simulink model "kalman_predictor"  (R2014a)
settings: Solver=FixedStepDiscrete  StartTime=0.0  StopTime=t_sim  FixedStep=t_step  RelTol=1e-3
undefined symbols (not defined in the file): omega_B
libraries: lib_gyro_fusion x3
settings Model: Creator=kirill  LastModifiedBy=kirill

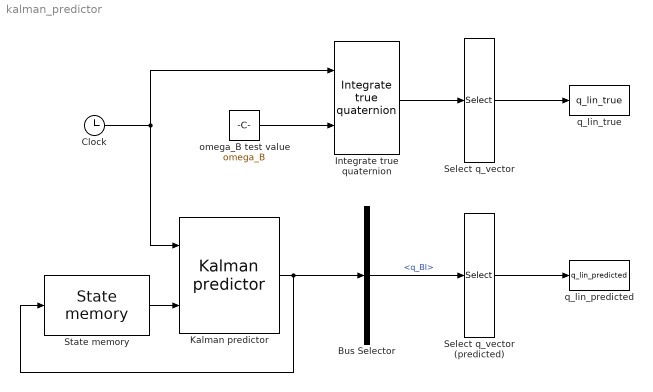
== system kalman_predictor ==
  Bus Selector : BusSelector  OutputSignals=q_BI
  Clock : Clock
  Integrate true quaternion : lib_gyro_fusion/Integrate true quaternion  q_BI_init=q_init
  Kalman predictor : lib_gyro_fusion/Kalman predictor  q_noise=0  omega_B_noise=[0, 0, 0]  omega_I_bias_noise=0
  Select q_vector : Selector  InputPortWidth=4  IndexOptions=Starting index (dialog)  Indices=2  OutputSizes=3
  Select q_vector (predicted) : Selector  InputPortWidth=4  IndexOptions=Starting index (dialog)  Indices=2  OutputSizes=3
  State memory : lib_gyro_fusion/State memory  q_BI_init=q_init  omega_B_init=omega_B  omega_I_bias_init=omega_bias_I  P_full_init=eye(9)
  omega_B test value : Constant  Value=omega_B
  q_lin_predicted : ToWorkspace  VariableName=q_lin_predicted  SaveFormat=Timeseries  SampleTime=-1
  q_lin_true : ToWorkspace  VariableName=q_lin_true  SaveFormat=Timeseries  SampleTime=-1
  wires:
  State memory/1 -> Kalman predictor/2
  Kalman predictor/1 -> Bus Selector/1, State memory/1
  Clock/1 -> Kalman predictor/1, Integrate true quaternion/1
  Integrate true quaternion/1 -> Select q_vector/1
  Bus Selector/1 -> Select q_vector (predicted)/1  "<q_BI>"
  Select q_vector/1 -> q_lin_true/1
  Select q_vector (predicted)/1 -> q_lin_predicted/1
  omega_B test value/1 -> Integrate true quaternion/2
